simulink model "RVG"  (R2023b)
settings: Solver=FixedStepAuto  StartTime=0.0  StopTime=3  FixedStep=0.005  RelTol=1e-3
undefined symbols (not defined in the file): DiscIntNeverNeededParam
settings Model: Creator=user  LastModifiedBy=user
settings OptimizationCC: DefaultParameterBehavior=Inlined  EnhancedBackFolding=on  PassReuseOutputArgsAs=Individual arguments  ZeroExternalMemoryAtStartup=off  ZeroInternalMemoryAtStartup=off  OptimizeBlockOrder=speed  DifferentSizesBufferReuse=on  OptimizationCustomize=off  EfficientTunableParamExpr=on
settings DebuggingCC: ParameterTunabilityLossMsg=error
settings SFSimCC: MATLABDynamicMemAlloc=off
settings RTWCC: Description=Embedded Coder  SystemTargetFile=ert.tlc  TemplateMakefile=ert_default_tmf
settings CodeAppCC: ForceParamTrailComments=on  IgnoreCustomStorageClasses=off  OperatorAnnotations=on  SimulinkDataObjDesc=on  SFDataObjDesc=on  InsertBlockDesc=on
settings ERTTargetCC: TargetLangStandard=C99 (ISO)  GenerateSampleERTMain=on  InlinedParameterPlacement=NonHierarchical  ERTCustomFileTemplate=example_file_process.tlc

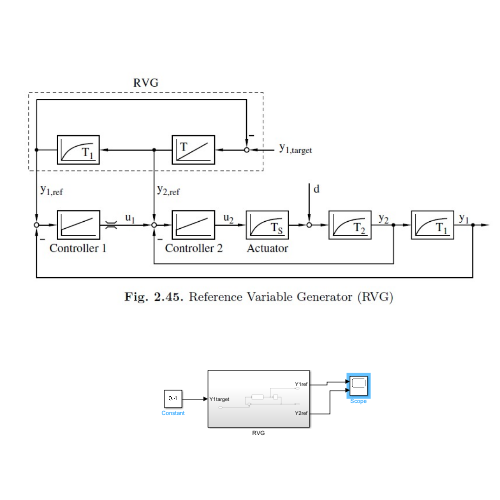
[thumbnail: Simulink's stored preview of the top-level diagram]
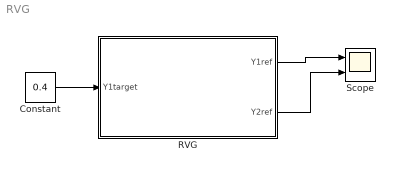
== system RVG ==
  Constant : Constant  Value=0.4
  RVG : Subsystem
  Scope : Scope  NumInputPorts=2
  wires:
  Constant/1 -> RVG/1(Y1target)
  RVG/1(Y1ref) -> Scope/1
  RVG/2(Y2ref) -> Scope/2

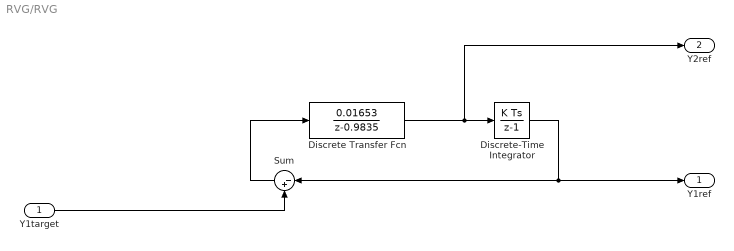
== system RVG/RVG ==
  Y1target : Inport
  Discrete Transfer Fcn : DiscreteTransferFcn  Numerator=[0.01653]  Denominator=[1 -0.9835]
  Discrete-Time Integrator : DiscreteIntegrator  SampleTime=-1  ICPrevOutput=DiscIntNeverNeededParam  ICPrevScaledInput=DiscIntNeverNeededParam
  Sum : Sum  Inputs=|-+
  Y1ref : Outport
  Y2ref : Outport  Port=2
  wires:
  Discrete Transfer Fcn/1 -> Discrete-Time Integrator/1, Y2ref/1
  Discrete-Time Integrator/1 -> Y1ref/1, Sum/1
  Sum/1 -> Discrete Transfer Fcn/1
  Y1target/1 -> Sum/2
